simulink model "Assignment_2"  (R2018a)
settings: Solver=VariableStepAuto  StartTime=0.0  StopTime=1  RelTol=1e-3
libraries: simulink x2, powerlib x1
settings Model: Creator=Aniket Raj  LastModifiedBy=Aniket Raj

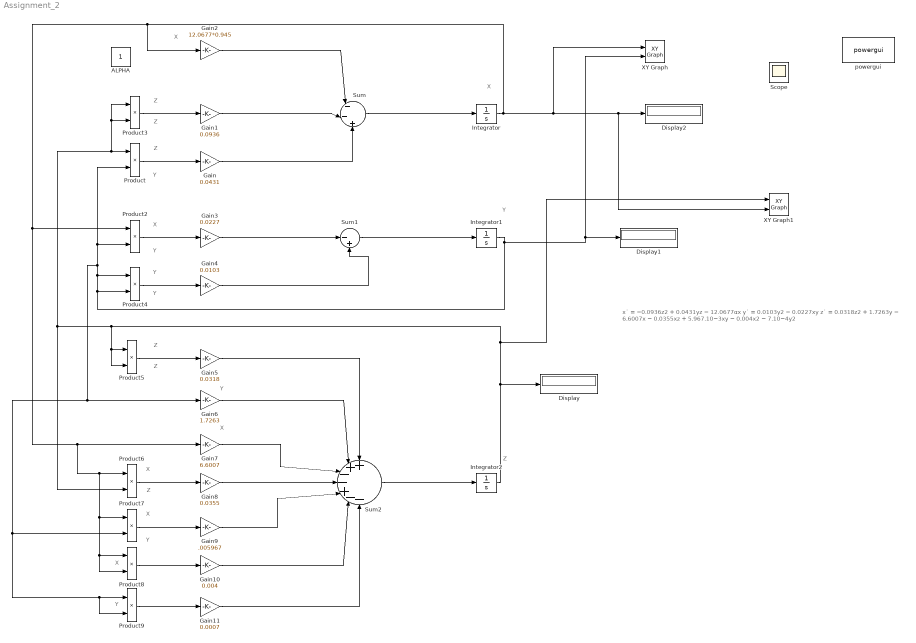
== system Assignment_2 ==
  note: x˙ = −0.0936z2 + 0.0431yz − 12.0677αx
      | y˙ = 0.0103y2 − 0.0227xy
      | z˙ = 0.0318z2 + 1.7263y − 6.6007x − 0.0355xz + 5.967.10−3xy − 0.004x2 − 7.10−4y2
  note: X
  note: Y
  note: Z
  note: Z
  note: Y
  note: Z
  note: X
  note: X
  note: Y
  note: Y
  note: Z
  note: Y
  note: X
  note: X
  note: Z
  note: Y
  note: X
  note: Y
  note: X
  note: Z
  note: Y
  note: Z
  ALPHA : Constant
  Display : Display
  Display1 : Display
  Display2 : Display
  Gain : Gain  Gain=0.0431
  Gain1 : Gain  Gain=0.0936
  Gain10 : Gain  Gain=0.004
  Gain11 : Gain  Gain=0.0007
  Gain2 : Gain  Gain=12.0677*0.945
  Gain3 : Gain  Gain=0.0227
  Gain4 : Gain  Gain=0.0103
  Gain5 : Gain  Gain=0.0318
  Gain6 : Gain  Gain=1.7263
  Gain7 : Gain  Gain=6.6007
  Gain8 : Gain  Gain=0.0355
  Gain9 : Gain  Gain=.005967
  Integrator : Integrator  InitialCondition=1
  Integrator1 : Integrator  InitialCondition=1
  Integrator2 : Integrator  InitialCondition=1
  Product{,2..9} (9 alike) : Product
  Scope : Scope
  Sum : Sum  Inputs=|-|-|+
  Sum1 : Sum  Inputs=|-+
  Sum2 : Sum  Inputs=+|+|-|-|+|-|-
  XY Graph : simulink/Sinks/XY Graph  xmin=-5  xmax=5  ymin=-5  ymax=5  st=0.01
  XY Graph1 : simulink/Sinks/XY Graph  xmin=-5  xmax=5  ymin=-5  ymax=5  st=0.01
  powergui : powerlib/powergui  Priority=1  SimulationMode=Continuous  SampleTime=50e-6  frequency=60  Iterations=50  frequencyindice=60  Pbase=100e6  ErrMax=1e-4  UnitsV=kV  UnitsW=MW  buscounter=0  FunctionMessages=off  echomessages=off  EnableUseOfTLC=off  CurrentSourceSwitches=off  DisableSnubberDevices=off  DisableRonSwitches=off  DisableVfSwitches=off  DisplayEquations=off  SolverType=Tustin/Backward Euler (TBE)  Interpol=off  ExternalGateDelay=off  methode=off  Ts=100  x0status=blocks  SPID=on  SwTol=0  HookPort=off  RestoreLinks=warning  ResistiveCurrentMeasurement=off  Frange=[0:2:500]  Ylog=off  Xlog=on  ShowGrid=off  save=off  variable=ZData  structure=0  ZoomFFT=off  StartTime=0.0  cycles=1  DisplayStyle=1  fundamental=60  FreqAxis=off  MaxFrequency=1000  frequencyindicesteady=1  RmsSteady=1  display=off
  wires:
  Sum/1 -> Integrator/1
  Sum1/1 -> Integrator1/1
  Sum2/1 -> Integrator2/1
  Gain/1 -> Sum/3
  Product/1 -> Gain/1
  Product3/1 -> Gain1/1
  Gain1/1 -> Sum/2
  Integrator/1 -> XY Graph/1, XY Graph1/2, Display2/1, Gain2/1, Product8/2, Product8/1, Product7/1, Product6/1, Gain7/1, Product2/1
  Gain2/1 -> Sum/1
  Product2/1 -> Gain3/1
  Gain3/1 -> Sum1/1
  Product4/1 -> Gain4/1
  Gain4/1 -> Sum1/2
  Product5/1 -> Gain5/1
  Gain5/1 -> Sum2/1
  Gain6/1 -> Sum2/2
  Gain7/1 -> Sum2/3
  Product6/1 -> Gain8/1
  Gain8/1 -> Sum2/4
  Product7/1 -> Gain9/1
  Gain9/1 -> Sum2/5
  Product8/1 -> Gain10/1
  Gain10/1 -> Sum2/6
  Product9/1 -> Gain11/1
  Gain11/1 -> Sum2/7
  Integrator2/1 -> Display/1, XY Graph1/1, Product3/1, Product3/2, Product/1, Product6/2, Product5/2, Product5/1
  Integrator1/1 -> XY Graph/2, Display1/1, Product4/2, Product4/1, Product9/2, Product9/1, Product7/2, Gain6/1, Product2/2, Product/2
